simulink model "case_2_ego0_gap_not_desired25a"  (R2025b)
settings: Solver=VariableStepAuto  StartTime=0.0  StopTime=10.0  RelTol=1e-3
settings Model: Creator=jdcjd  LastModifiedBy=admin

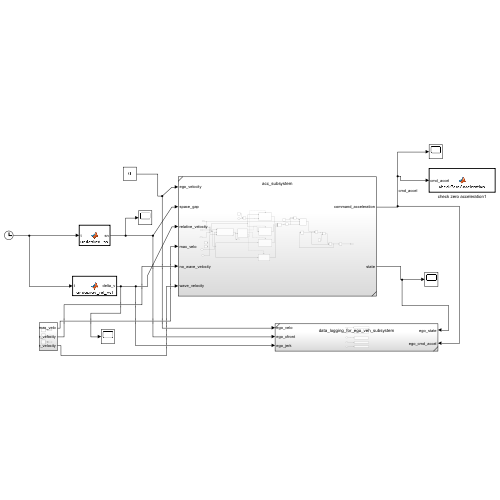
[thumbnail: Simulink's stored preview of the top-level diagram]
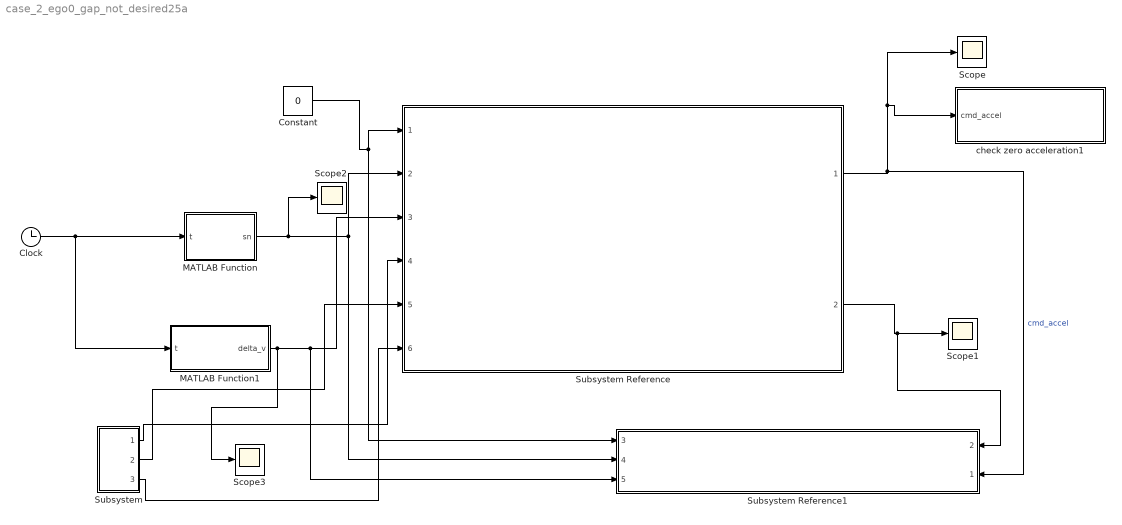
== system case_2_ego0_gap_not_desired25a ==
  Clock : Clock
  Constant : Constant  Value=0
  MATLAB Function : MATLAB Function  TreatAsAtomicUnit=on
  MATLAB Function1 : MATLAB Function  TreatAsAtomicUnit=on
  Scope{,1..3} (4 alike) : Scope
      Scope settings: ActiveDisplayYMinimum=-0.16874999999999998  ActiveDisplayYMaximum=1.51875
      Scope1 settings: ActiveDisplayYMinimum=-0.37499999999999989  ActiveDisplayYMaximum=3.375
      Scope2 settings: ActiveDisplayYMinimum=-0.17568020408606511  ActiveDisplayYMaximum=1.1266479209139351  DataLoggingVariableName=ScopeData2
      Scope3 settings: ActiveDisplayYMinimum=-0.62499999999999989  ActiveDisplayYMaximum=5.625  DataLoggingVariableName=ScopeData3
  Subsystem : Subsystem
  Subsystem Reference : Subsystem  ReferencedSubsystem=acc_subsystem
  Subsystem Reference1 : Subsystem  ReferencedSubsystem=data_logging_for_ego_veh_subsystem
      settings: PortSchema="{\"entries\":[{\"content\":{\"sides\":[{\"content\":{\"connectorIds\":[\"In3\",\"In4\",\"In5\"]},\"type\":\"ConnectorPlacement.EquallySpacedRectSide\",\"uuid\":\"0b96bcaa-a470-46c9-9268-f4bd6b1035a8\"},{\"content\":{\"connectorIds\":[\"In2\",\"In1\"],\"side\":\"RIGHT\"},\"type\":\"ConnectorPlacement.EquallySpacedRectSide\",\"uuid\":\"8e49005a-1e53-4e76-b163-50df0eb9f2cc\"},{\"content\":{\"side\":\"TOP\"},\"type\":\"ConnectorPlacement.EquallySpacedRectSide\",\"uuid\":\"3ff4af65-efca-4a64-9b7f-f479498e89e2\"}]},\"type\":\"ConnectorPlacement.EquallySpacedConnector\",\"uuid\":\"f10caef7-9599-4d5c-a8fd-3eb49f6fcaa8\"}],\"packageUris\":[\"http://schema.mathworks.com/mf0/Connector/R2020b\"],\"version\":\"1.0\"}"
  check zero acceleration1 : MATLAB Function  TreatAsAtomicUnit=on
  wires:
  Subsystem Reference/2 -> Subsystem Reference1/2, Scope1/1
  MATLAB Function/1(sn) -> Scope2/1, Subsystem Reference1/4, Subsystem Reference/2
  Clock/1 -> MATLAB Function1/1(t), MATLAB Function/1(t)
  MATLAB Function1/1(delta_v) -> Scope3/1, Subsystem Reference1/5, Subsystem Reference/3
  Subsystem Reference/1 -> Subsystem Reference1/1, check zero acceleration1/1(cmd_accel), Scope/1  "cmd_accel"
  Constant/1 -> Subsystem Reference1/3, Subsystem Reference/1
  Subsystem/2(no_wave_velocity) -> Subsystem Reference/5
  Subsystem/1(max_velo) -> Subsystem Reference/4
  Subsystem/3(wave_velocity) -> Subsystem Reference/6

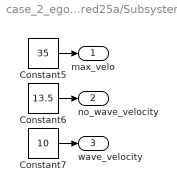
== system case_2_ego0_gap_not_desired25a/Subsystem ==
  Constant5 : Constant  Value=35
  Constant6 : Constant  Value=13.5
  Constant7 : Constant  Value=10
  max_velo : Outport
  no_wave_velocity : Outport  Port=2
  wave_velocity : Outport  Port=3
  wires:
  Constant7/1 -> wave_velocity/1
  Constant6/1 -> no_wave_velocity/1
  Constant5/1 -> max_velo/1

== matlab function case_2_ego0_gap_not_desired25a/MATLAB Function ==
  data: t input; sn output
function sn = undesired_sn(t)

sn = min(t, 0.9);
end

== matlab function case_2_ego0_gap_not_desired25a/check zero acceleration1 ==
  data: cmd_accel input
function checkZeroAcceleration(cmd_accel)
%#codegen
coder.extrinsic('disp', 'sprintf');

if cmd_accel > 0
    msg = sprintf('Error: non zero command acceleration: %.3f, should be less or equal zero', ...
                  cmd_accel);
    disp(msg);
end
end

== matlab function case_2_ego0_gap_not_desired25a/MATLAB Function1 ==
  data: t input; delta_v output
function delta_v = undesired_rel_vel(t)

delta_v = min(t, 5);
end
